simulink model "simul_task3"  (R2021b)
settings: Solver=FixedStepAuto  StartTime=0.0  StopTime=10.0  FixedStep=10e-5  RelTol=1e-3
undefined symbols (not defined in the file): A, B, C, D, I
libraries: fuzblock x1
settings Model: Creator=witold  LastModifiedBy=witold

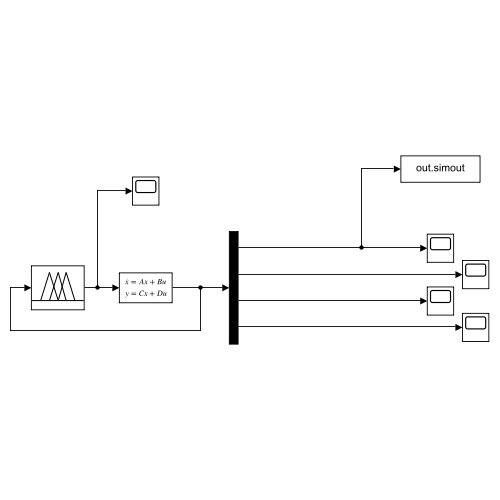
[thumbnail: Simulink's stored preview of the top-level diagram]
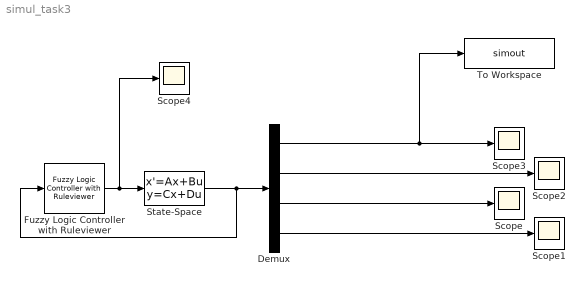
== system simul_task3 ==
  Demux : Demux
  Fuzzy Logic Controller with Ruleviewer : fuzblock/Fuzzy Logic  Controller  with Ruleviewer  fismatrix=fuzzy1  Ts=2
  Scope{,1..4} (5 alike) : Scope
  State-Space : StateSpace  A=A  B=B  C=C  D=D  InitialCondition=I  ContinuousStateAttributes={'theta','theta_dot','x','x_dot'}
  To Workspace : ToWorkspace  VariableName=simout  SampleTime=-1
  wires:
  Fuzzy Logic Controller with Ruleviewer/1 -> Scope4/1, State-Space/1
  State-Space/1 -> Fuzzy Logic Controller with Ruleviewer/1, Demux/1
  Demux/1 -> To Workspace/1, Scope3/1
  Demux/2 -> Scope2/1
  Demux/3 -> Scope/1
  Demux/4 -> Scope1/1
